simulink model "SIMULINK"  (R2020b)
settings: Solver=ode45  StartTime=0.0  StopTime=100  RelTol=1e-3
values from neighbouring files (symbols this model uses):
  beta = 0.4    [RGT4.m]    (also in RGTSS.m = param(1))
  Do = 0    [RGT4.m]    (also in RGTSS.m)
  gamma = 0.035    [RGT4.m]    (also in RGTSS.m = param(2))
  Io = 3    [RGT4.m]    (also in RGTSS.m)
  mu = 0.005    [RGT4.m]    (also in RGTSS.m = param(3))
  N = 580000    [NC_DATA.m]    (also in RGT4.m = 1000; RGTSS.m)
  Ro = 0    [RGT4.m]    (also in RGTSS.m)
  So = 997    [RGT4.m]    (also in RGTSS.m = 579997)
settings Model: Creator=Gabriel Andre  LastModifiedBy=Gabriel Andre

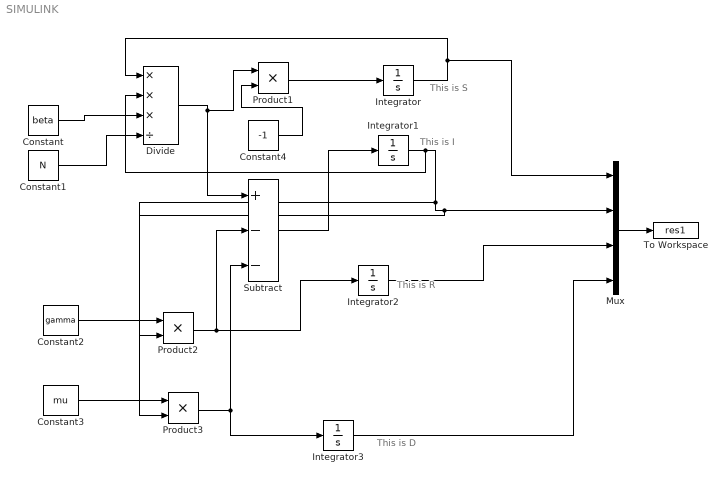
== system SIMULINK ==
  note: This is D
  note: This is R
  note: This is I
  note: This is S
  Constant : Constant  Value=beta
  Constant1 : Constant  Value=N
  Constant2 : Constant  Value=gamma
  Constant3 : Constant  Value=mu
  Constant4 : Constant  Value=-1
  Divide : Product  Inputs=***/
  Integrator : Integrator  InitialCondition=So
  Integrator1 : Integrator  InitialCondition=Io
  Integrator2 : Integrator  InitialCondition=Ro
  Integrator3 : Integrator  InitialCondition=Do
  Mux : Mux
  Product1 : Product
  Product2 : Product
  Product3 : Product
  Subtract : Sum  Inputs=+--
  To Workspace : ToWorkspace  VariableName=res1  SaveFormat=Structure With Time  SampleTime=-1
  wires:
  Integrator/1 -> Divide/1, Mux/1
  Integrator1/1 -> Divide/2, Product3/2, Product2/2, Mux/2
  Integrator2/1 -> Mux/3
  Integrator3/1 -> Mux/4
  Constant1/1 -> Divide/4
  Constant4/1 -> Product1/2
  Divide/1 -> Subtract/1, Product1/1
  Product1/1 -> Integrator/1
  Constant2/1 -> Product2/1
  Constant3/1 -> Product3/1
  Subtract/1 -> Integrator1/1
  Product2/1 -> Integrator2/1, Subtract/2
  Product3/1 -> Integrator3/1, Subtract/3
  Constant/1 -> Divide/3
  Mux/1 -> To Workspace/1
